simulink model "AutonomousCleaningSystem"  (R2022b)
settings: Solver=VariableStepAuto  StartTime=0.0  StopTime=10.0  RelTol=1e-3
undefined symbols (not defined in the file): Camera_data, Lidar
settings Model: Creator=carol  LastModifiedBy=carol
settings OptimizationCC: ReuseModelBlockBuffer=on

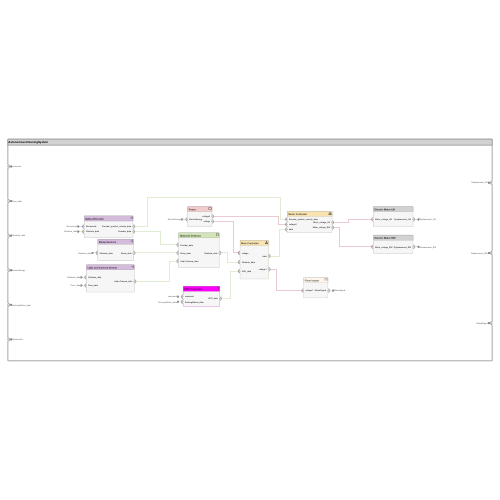
[thumbnail: Simulink's stored preview of the top-level diagram]
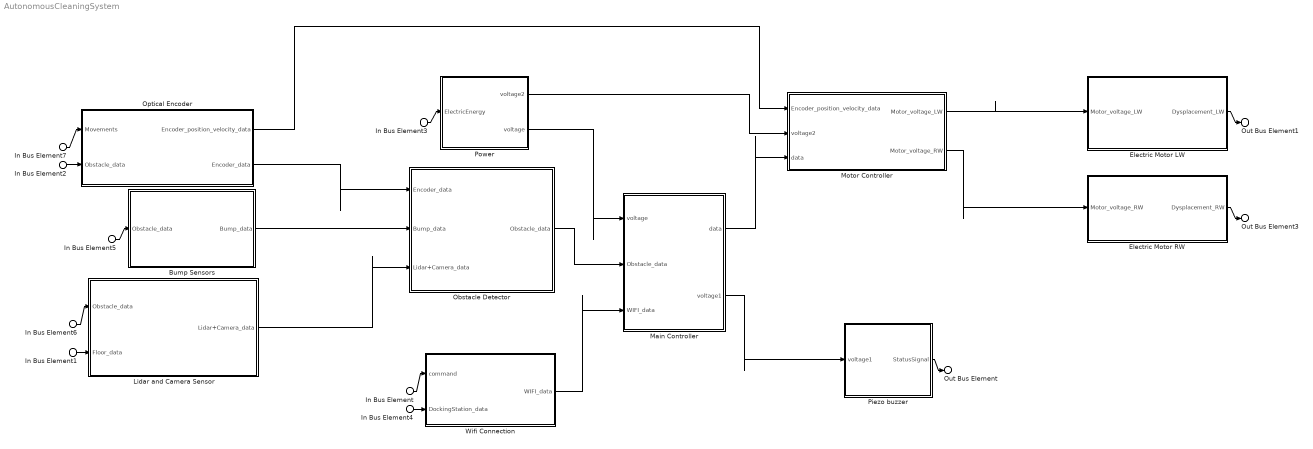
== system AutonomousCleaningSystem ==
  In Bus Element : Inport  PortName=command
  In Bus Element1 : Inport  Port=2  PortName=Floor_data
  In Bus Element2 : Inport  Port=3  PortName=Obstacle_data
  In Bus Element5 : Inport  Port=3  PortName=Obstacle_data
  In Bus Element6 : Inport  Port=3  PortName=Obstacle_data
  In Bus Element3 : Inport  Port=4  PortName=ElectricEnergy
  In Bus Element4 : Inport  Port=5  PortName=DockingStation_data
  In Bus Element7 : Inport  Port=6  PortName=Movements
  Bump Sensors : Subsystem
      settings: PortSchema="{\"entries\":[{\"content\":{\"headerSize\":26,\"margin\":15,\"minimumSpacing\":25,\"sides\":[{\"content\":{\"connectorIds\":[\"In1\"]},\"type\":\"ConnectorPlacement.EquallySpacedRectSide\",\"uuid\":\"6ae6270c-bff4-4a0d-8fba-8fdec87b0a05\"},{\"content\":{\"connectorIds\":[\"Out1\"],\"side\":\"RIGHT\"},\"type\":\"ConnectorPlacement.EquallySpacedRectSide\",\"uuid\":\"f3a0045b-bb3b-40f9-afd5-e1537ff3eeca\"},{\"content\":{\"side\":\"TOP\"},\"type\":\"ConnectorPlacement.EquallySpacedRectSide\",\"uuid\":\"e89a58f2-90b0-468c-bb6a-95617af68e24\"}]},\"type\":\"ConnectorPlacement.EquallySpacedConnector\",\"uuid\":\"066eb43c-7b96-4660-9f29-628dd77a5b3b\"}],\"packageUris\":[\"http://schema.mathworks.com/mf0/Connector/R2020b\"],\"version\":\"1.0\"}"
  Electric Motor LW : Subsystem
      settings: PortSchema="{\"entries\":[{\"content\":{\"headerSize\":26,\"margin\":15,\"minimumSpacing\":25,\"sides\":[{\"content\":{\"connectorIds\":[\"In1\"]},\"type\":\"ConnectorPlacement.EquallySpacedRectSide\",\"uuid\":\"6ae6270c-bff4-4a0d-8fba-8fdec87b0a05\"},{\"content\":{\"connectorIds\":[\"Out1\"],\"side\":\"RIGHT\"},\"type\":\"ConnectorPlacement.EquallySpacedRectSide\",\"uuid\":\"f3a0045b-bb3b-40f9-afd5-e1537ff3eeca\"},{\"content\":{\"side\":\"TOP\"},\"type\":\"ConnectorPlacement.EquallySpacedRectSide\",\"uuid\":\"e89a58f2-90b0-468c-bb6a-95617af68e24\"}]},\"type\":\"ConnectorPlacement.EquallySpacedConnector\",\"uuid\":\"066eb43c-7b96-4660-9f29-628dd77a5b3b\"}],\"packageUris\":[\"http://schema.mathworks.com/mf0/Connector/R2020b\"],\"version\":\"1.0\"}"
  Electric Motor RW : Subsystem
      settings: PortSchema="{\"entries\":[{\"content\":{\"headerSize\":26,\"margin\":15,\"minimumSpacing\":25,\"sides\":[{\"content\":{\"connectorIds\":[\"In1\"]},\"type\":\"ConnectorPlacement.EquallySpacedRectSide\",\"uuid\":\"6ae6270c-bff4-4a0d-8fba-8fdec87b0a05\"},{\"content\":{\"connectorIds\":[\"Out1\"],\"side\":\"RIGHT\"},\"type\":\"ConnectorPlacement.EquallySpacedRectSide\",\"uuid\":\"f3a0045b-bb3b-40f9-afd5-e1537ff3eeca\"},{\"content\":{\"side\":\"TOP\"},\"type\":\"ConnectorPlacement.EquallySpacedRectSide\",\"uuid\":\"e89a58f2-90b0-468c-bb6a-95617af68e24\"}]},\"type\":\"ConnectorPlacement.EquallySpacedConnector\",\"uuid\":\"066eb43c-7b96-4660-9f29-628dd77a5b3b\"}],\"packageUris\":[\"http://schema.mathworks.com/mf0/Connector/R2020b\"],\"version\":\"1.0\"}"
  Lidar and Camera Sensor : Subsystem
      settings: PortSchema="{\"entries\":[{\"content\":{\"headerSize\":26,\"margin\":15,\"minimumSpacing\":25,\"sides\":[{\"content\":{\"connectorIds\":[\"In1\",\"In2\"]},\"type\":\"ConnectorPlacement.EquallySpacedRectSide\",\"uuid\":\"6ae6270c-bff4-4a0d-8fba-8fdec87b0a05\"},{\"content\":{\"connectorIds\":[\"Out1\"],\"side\":\"RIGHT\"},\"type\":\"ConnectorPlacement.EquallySpacedRectSide\",\"uuid\":\"f3a0045b-bb3b-40f9-afd5-e1537ff3eeca\"},{\"content\":{\"side\":\"TOP\"},\"type\":\"ConnectorPlacement.EquallySpacedRectSide\",\"uuid\":\"e89a58f2-90b0-468c-bb6a-95617af68e24\"}]},\"type\":\"ConnectorPlacement.EquallySpacedConnector\",\"uuid\":\"066eb43c-7b96-4660-9f29-628dd77a5b3b\"}],\"packageUris\":[\"http://schema.mathworks.com/mf0/Connector/R2020b\"],\"version\":\"1.0\"}"
  Main Controller : Subsystem
      settings: PortSchema="{\"entries\":[{\"content\":{\"headerSize\":26,\"margin\":15,\"minimumSpacing\":25,\"sides\":[{\"content\":{\"connectorIds\":[\"In1\",\"In2\",\"In3\"]},\"type\":\"ConnectorPlacement.EquallySpacedRectSide\",\"uuid\":\"6ae6270c-bff4-4a0d-8fba-8fdec87b0a05\"},{\"content\":{\"connectorIds\":[\"Out1\",\"Out2\"],\"side\":\"RIGHT\"},\"type\":\"ConnectorPlacement.EquallySpacedRectSide\",\"uuid\":\"f3a0045b-bb3b-40f9-afd5-e1537ff3eeca\"},{\"content\":{\"side\":\"TOP\"},\"type\":\"ConnectorPlacement.EquallySpacedRectSide\",\"uuid\":\"e89a58f2-90b0-468c-bb6a-95617af68e24\"}]},\"type\":\"ConnectorPlacement.EquallySpacedConnector\",\"uuid\":\"066eb43c-7b96-4660-9f29-628dd77a5b3b\"}],\"packageUris\":[\"http://schema.mathworks.com/mf0/Connector/R2020b\"],\"version\":\"1.0\"}"
  Motor Controller : Subsystem
      settings: PortSchema="{\"entries\":[{\"content\":{\"headerSize\":26,\"margin\":15,\"minimumSpacing\":25,\"sides\":[{\"content\":{\"connectorIds\":[\"In1\",\"In2\",\"In3\"]},\"type\":\"ConnectorPlacement.EquallySpacedRectSide\",\"uuid\":\"6ae6270c-bff4-4a0d-8fba-8fdec87b0a05\"},{\"content\":{\"connectorIds\":[\"Out1\",\"Out2\"],\"side\":\"RIGHT\"},\"type\":\"ConnectorPlacement.EquallySpacedRectSide\",\"uuid\":\"f3a0045b-bb3b-40f9-afd5-e1537ff3eeca\"},{\"content\":{\"side\":\"TOP\"},\"type\":\"ConnectorPlacement.EquallySpacedRectSide\",\"uuid\":\"e89a58f2-90b0-468c-bb6a-95617af68e24\"}]},\"type\":\"ConnectorPlacement.EquallySpacedConnector\",\"uuid\":\"066eb43c-7b96-4660-9f29-628dd77a5b3b\"}],\"packageUris\":[\"http://schema.mathworks.com/mf0/Connector/R2020b\"],\"version\":\"1.0\"}"
  Obstacle Detector : Subsystem
      settings: PortSchema="{\"entries\":[{\"content\":{\"headerSize\":26,\"margin\":15,\"minimumSpacing\":25,\"sides\":[{\"content\":{\"connectorIds\":[\"In1\",\"In2\",\"In3\"]},\"type\":\"ConnectorPlacement.EquallySpacedRectSide\",\"uuid\":\"6ae6270c-bff4-4a0d-8fba-8fdec87b0a05\"},{\"content\":{\"connectorIds\":[\"Out1\"],\"side\":\"RIGHT\"},\"type\":\"ConnectorPlacement.EquallySpacedRectSide\",\"uuid\":\"f3a0045b-bb3b-40f9-afd5-e1537ff3eeca\"},{\"content\":{\"side\":\"TOP\"},\"type\":\"ConnectorPlacement.EquallySpacedRectSide\",\"uuid\":\"e89a58f2-90b0-468c-bb6a-95617af68e24\"}]},\"type\":\"ConnectorPlacement.EquallySpacedConnector\",\"uuid\":\"066eb43c-7b96-4660-9f29-628dd77a5b3b\"}],\"packageUris\":[\"http://schema.mathworks.com/mf0/Connector/R2020b\"],\"version\":\"1.0\"}"
  Optical Encoder : Subsystem
      settings: PortSchema="{\"entries\":[{\"content\":{\"headerSize\":26,\"margin\":15,\"minimumSpacing\":25,\"sides\":[{\"content\":{\"connectorIds\":[\"In1\",\"In2\"]},\"type\":\"ConnectorPlacement.EquallySpacedRectSide\",\"uuid\":\"6ae6270c-bff4-4a0d-8fba-8fdec87b0a05\"},{\"content\":{\"connectorIds\":[\"Out1\",\"Out2\"],\"side\":\"RIGHT\"},\"type\":\"ConnectorPlacement.EquallySpacedRectSide\",\"uuid\":\"f3a0045b-bb3b-40f9-afd5-e1537ff3eeca\"},{\"content\":{\"side\":\"TOP\"},\"type\":\"ConnectorPlacement.EquallySpacedRectSide\",\"uuid\":\"e89a58f2-90b0-468c-bb6a-95617af68e24\"}]},\"type\":\"ConnectorPlacement.EquallySpacedConnector\",\"uuid\":\"066eb43c-7b96-4660-9f29-628dd77a5b3b\"}],\"packageUris\":[\"http://schema.mathworks.com/mf0/Connector/R2020b\"],\"version\":\"1.0\"}"
  Piezo buzzer : Subsystem
      settings: PortSchema="{\"entries\":[{\"content\":{\"headerSize\":26,\"margin\":15,\"minimumSpacing\":25,\"sides\":[{\"content\":{\"connectorIds\":[\"In1\"]},\"type\":\"ConnectorPlacement.EquallySpacedRectSide\",\"uuid\":\"6ae6270c-bff4-4a0d-8fba-8fdec87b0a05\"},{\"content\":{\"connectorIds\":[\"Out1\"],\"side\":\"RIGHT\"},\"type\":\"ConnectorPlacement.EquallySpacedRectSide\",\"uuid\":\"f3a0045b-bb3b-40f9-afd5-e1537ff3eeca\"},{\"content\":{\"side\":\"TOP\"},\"type\":\"ConnectorPlacement.EquallySpacedRectSide\",\"uuid\":\"e89a58f2-90b0-468c-bb6a-95617af68e24\"}]},\"type\":\"ConnectorPlacement.EquallySpacedConnector\",\"uuid\":\"066eb43c-7b96-4660-9f29-628dd77a5b3b\"}],\"packageUris\":[\"http://schema.mathworks.com/mf0/Connector/R2020b\"],\"version\":\"1.0\"}"
  Power : Subsystem
      settings: PortSchema="{\"entries\":[{\"content\":{\"headerSize\":26,\"margin\":15,\"minimumSpacing\":25,\"sides\":[{\"content\":{\"connectorIds\":[\"In1\"]},\"type\":\"ConnectorPlacement.EquallySpacedRectSide\",\"uuid\":\"6ae6270c-bff4-4a0d-8fba-8fdec87b0a05\"},{\"content\":{\"connectorIds\":[\"Out2\",\"Out1\"],\"side\":\"RIGHT\"},\"type\":\"ConnectorPlacement.EquallySpacedRectSide\",\"uuid\":\"f3a0045b-bb3b-40f9-afd5-e1537ff3eeca\"},{\"content\":{\"side\":\"TOP\"},\"type\":\"ConnectorPlacement.EquallySpacedRectSide\",\"uuid\":\"e89a58f2-90b0-468c-bb6a-95617af68e24\"}]},\"type\":\"ConnectorPlacement.EquallySpacedConnector\",\"uuid\":\"066eb43c-7b96-4660-9f29-628dd77a5b3b\"}],\"packageUris\":[\"http://schema.mathworks.com/mf0/Connector/R2020b\"],\"version\":\"1.0\"}"
  Wifi Connection : Subsystem
      settings: PortSchema="{\"entries\":[{\"content\":{\"headerSize\":26,\"margin\":15,\"minimumSpacing\":25,\"sides\":[{\"content\":{\"connectorIds\":[\"In2\",\"In1\"]},\"type\":\"ConnectorPlacement.EquallySpacedRectSide\",\"uuid\":\"6ae6270c-bff4-4a0d-8fba-8fdec87b0a05\"},{\"content\":{\"connectorIds\":[\"Out1\"],\"side\":\"RIGHT\"},\"type\":\"ConnectorPlacement.EquallySpacedRectSide\",\"uuid\":\"f3a0045b-bb3b-40f9-afd5-e1537ff3eeca\"},{\"content\":{\"side\":\"TOP\"},\"type\":\"ConnectorPlacement.EquallySpacedRectSide\",\"uuid\":\"e89a58f2-90b0-468c-bb6a-95617af68e24\"}]},\"type\":\"ConnectorPlacement.EquallySpacedConnector\",\"uuid\":\"066eb43c-7b96-4660-9f29-628dd77a5b3b\"}],\"packageUris\":[\"http://schema.mathworks.com/mf0/Connector/R2020b\"],\"version\":\"1.0\"}"
  Out Bus Element1 : Outport  PortName=Displacement_LW
  Out Bus Element3 : Outport  Port=2  PortName=Displacement_RW
  Out Bus Element : Outport  Port=3  PortName=StatusSignal
  wires:
  In Bus Element4/1 -> Wifi Connection/1(DockingStation_data)
  Obstacle Detector/1(Obstacle_data) -> Main Controller/2(Obstacle_data)
  Electric Motor LW/1(Dysplacement_LW) -> Out Bus Element1/1
  Piezo buzzer/1(StatusSignal) -> Out Bus Element/1
  In Bus Element1/1 -> Lidar and Camera Sensor/2(Floor_data)
  Electric Motor RW/1(Dysplacement_RW) -> Out Bus Element3/1
  Wifi Connection/1(WIFI_data) -> Main Controller/3(WIFI_data)
  In Bus Element7/1 -> Optical Encoder/1(Movements)
  Motor Controller/2(Motor_voltage_RW) -> Electric Motor RW/1(Motor_voltage_RW)
  In Bus Element/1 -> Wifi Connection/2(command)
  Power/1(voltage) -> Main Controller/1(voltage)
  In Bus Element3/1 -> Power/1(ElectricEnergy)
  In Bus Element2/1 -> Optical Encoder/2(Obstacle_data)
  Optical Encoder/2(Encoder_data) -> Obstacle Detector/1(Encoder_data)
  Main Controller/2(voltage1) -> Piezo buzzer/1(voltage1)
  Motor Controller/1(Motor_voltage_LW) -> Electric Motor LW/1(Motor_voltage_LW)
  In Bus Element6/1 -> Lidar and Camera Sensor/1(Obstacle_data)
  In Bus Element5/1 -> Bump Sensors/1(Obstacle_data)
  Main Controller/1(data) -> Motor Controller/3(data)
  Optical Encoder/1(Encoder_position_velocity_data) -> Motor Controller/1(Encoder_position_velocity_data)
  Bump Sensors/1(Bump_data) -> Obstacle Detector/2(Bump_data)
  Lidar and Camera Sensor/1(Lidar+Camera_data) -> Obstacle Detector/3(Lidar+Camera_data)
  Power/2(voltage2) -> Motor Controller/2(voltage2)

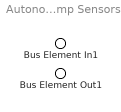
== system AutonomousCleaningSystem/Bump Sensors ==
  Bus Element In1 : Inport  PortName=Obstacle_data
  Bus Element Out1 : Outport  PortName=Bump_data

== system AutonomousCleaningSystem/Electric Motor LW ==
  Bus Element In1 : Inport  PortName=Motor_voltage_LW
  Bus Element Out1 : Outport  PortName=Dysplacement_LW

== system AutonomousCleaningSystem/Electric Motor RW ==
  Bus Element In1 : Inport  PortName=Motor_voltage_RW
  Bus Element Out1 : Outport  PortName=Dysplacement_RW

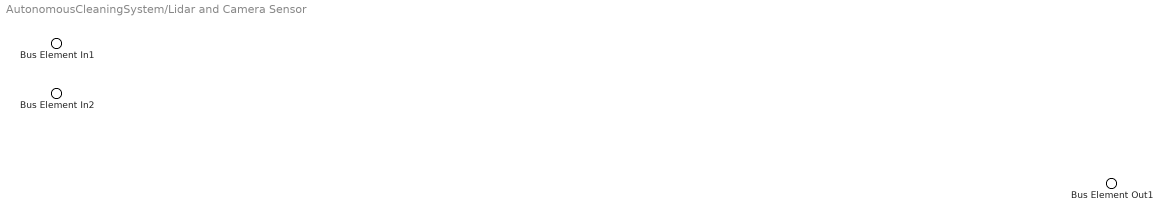
== system AutonomousCleaningSystem/Lidar and Camera Sensor ==
  Bus Element In1 : Inport  PortName=Obstacle_data
  Bus Element In2 : Inport  Port=2  PortName=Floor_data
  Bus Element Out1 : Outport  PortName=Lidar+Camera_data

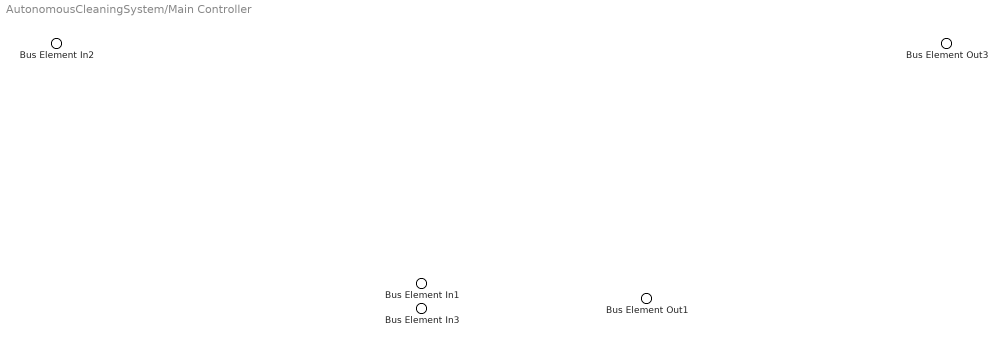
== system AutonomousCleaningSystem/Main Controller ==
  Bus Element In2 : Inport  PortName=voltage
  Bus Element In1 : Inport  Port=2  PortName=Obstacle_data
  Bus Element In3 : Inport  Port=3  PortName=WIFI_data
  Bus Element Out1 : Outport  PortName=data
  Bus Element Out3 : Outport  Port=2  PortName=voltage1

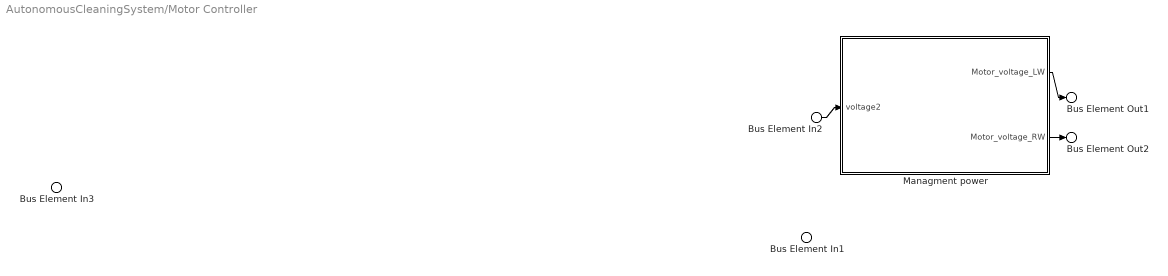
== system AutonomousCleaningSystem/Motor Controller ==
  Bus Element In3 : Inport  PortName=Encoder_position_velocity_data
  Bus Element In2 : Inport  Port=2  PortName=voltage2
  Bus Element In1 : Inport  Port=3  PortName=data
  Managment power : Subsystem
      settings: PortSchema="{\"entries\":[{\"content\":{\"headerSize\":26,\"margin\":15,\"minimumSpacing\":25,\"sides\":[{\"content\":{\"connectorIds\":[\"In1\"]},\"type\":\"ConnectorPlacement.EquallySpacedRectSide\",\"uuid\":\"8bc022de-dffb-4362-a5f8-17ef95234df5\"},{\"content\":{\"connectorIds\":[\"Out1\",\"Out2\"],\"side\":\"RIGHT\"},\"type\":\"ConnectorPlacement.EquallySpacedRectSide\",\"uuid\":\"7821fee0-4f8e-4fbb-ae89-26aabe366038\"},{\"content\":{\"side\":\"TOP\"},\"type\":\"ConnectorPlacement.EquallySpacedRectSide\",\"uuid\":\"eaa51f63-b7e5-4e12-92d3-5116fe88bdcc\"}]},\"type\":\"ConnectorPlacement.EquallySpacedConnector\",\"uuid\":\"a20c8fba-198d-4ab4-9322-4dfa42a9e59c\"}],\"packageUris\":[\"http://schema.mathworks.com/mf0/Connector/R2020b\"],\"version\":\"1.0\"}"
  Bus Element Out1 : Outport  PortName=Motor_voltage_LW
  Bus Element Out2 : Outport  Port=2  PortName=Motor_voltage_RW
  wires:
  Bus Element In2/1 -> Managment power/1(voltage2)
  Managment power/1(Motor_voltage_LW) -> Bus Element Out1/1
  Managment power/2(Motor_voltage_RW) -> Bus Element Out2/1

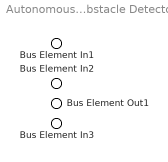
== system AutonomousCleaningSystem/Obstacle Detector ==
  Bus Element In1 : Inport  PortName=Encoder_data
  Bus Element In2 : Inport  Port=2  PortName=Bump_data
  Bus Element In3 : Inport  Port=3  PortName=Lidar+Camera_data
  Bus Element Out1 : Outport  PortName=Obstacle_data

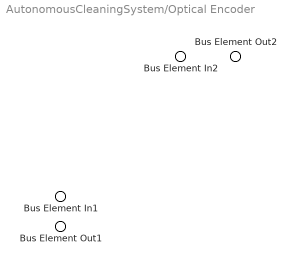
== system AutonomousCleaningSystem/Optical Encoder ==
  Bus Element In2 : Inport  PortName=Movements
  Bus Element In1 : Inport  Port=2  PortName=Obstacle_data
  Bus Element Out2 : Outport  PortName=Encoder_position_velocity_data
  Bus Element Out1 : Outport  Port=2  PortName=Encoder_data

== system AutonomousCleaningSystem/Piezo buzzer ==
  Bus Element In1 : Inport  PortName=voltage1
  Bus Element Out1 : Outport  PortName=StatusSignal

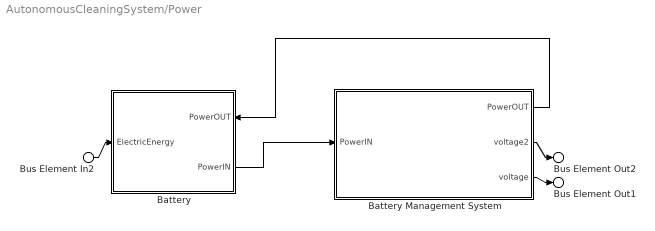
== system AutonomousCleaningSystem/Power ==
  Bus Element In2 : Inport  PortName=ElectricEnergy
  Battery : Subsystem
      settings: PortSchema="{\"entries\":[{\"content\":{\"headerSize\":26,\"margin\":15,\"minimumSpacing\":25,\"sides\":[{\"content\":{\"connectorIds\":[\"In2\"]},\"type\":\"ConnectorPlacement.EquallySpacedRectSide\",\"uuid\":\"8bc022de-dffb-4362-a5f8-17ef95234df5\"},{\"content\":{\"connectorIds\":[\"In1\",\"Out1\"],\"side\":\"RIGHT\"},\"type\":\"ConnectorPlacement.EquallySpacedRectSide\",\"uuid\":\"7821fee0-4f8e-4fbb-ae89-26aabe366038\"},{\"content\":{\"side\":\"TOP\"},\"type\":\"ConnectorPlacement.EquallySpacedRectSide\",\"uuid\":\"eaa51f63-b7e5-4e12-92d3-5116fe88bdcc\"}]},\"type\":\"ConnectorPlacement.EquallySpacedConnector\",\"uuid\":\"a20c8fba-198d-4ab4-9322-4dfa42a9e59c\"}],\"packageUris\":[\"http://schema.mathworks.com/mf0/Connector/R2020b\"],\"version\":\"1.0\"}"
  Battery Management System : Subsystem
      settings: PortSchema="{\"entries\":[{\"content\":{\"headerSize\":26,\"margin\":15,\"minimumSpacing\":25,\"sides\":[{\"content\":{\"connectorIds\":[\"In1\"]},\"type\":\"ConnectorPlacement.EquallySpacedRectSide\",\"uuid\":\"8bc022de-dffb-4362-a5f8-17ef95234df5\"},{\"content\":{\"connectorIds\":[\"Out1\",\"Out2\",\"Out3\"],\"side\":\"RIGHT\"},\"type\":\"ConnectorPlacement.EquallySpacedRectSide\",\"uuid\":\"7821fee0-4f8e-4fbb-ae89-26aabe366038\"},{\"content\":{\"side\":\"TOP\"},\"type\":\"ConnectorPlacement.EquallySpacedRectSide\",\"uuid\":\"eaa51f63-b7e5-4e12-92d3-5116fe88bdcc\"}]},\"type\":\"ConnectorPlacement.EquallySpacedConnector\",\"uuid\":\"a20c8fba-198d-4ab4-9322-4dfa42a9e59c\"}],\"packageUris\":[\"http://schema.mathworks.com/mf0/Connector/R2020b\"],\"version\":\"1.0\"}"
  Bus Element Out1 : Outport  PortName=voltage
  Bus Element Out2 : Outport  Port=2  PortName=voltage2
  wires:
  Battery/1(PowerIN) -> Battery Management System/1(PowerIN)
  Bus Element In2/1 -> Battery/2(ElectricEnergy)
  Battery Management System/1(PowerOUT) -> Battery/1(PowerOUT)
  Battery Management System/2(voltage2) -> Bus Element Out2/1
  Battery Management System/3(voltage) -> Bus Element Out1/1

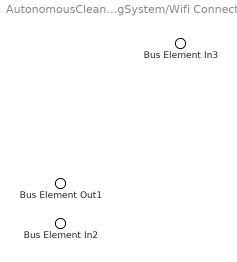
== system AutonomousCleaningSystem/Wifi Connection ==
  Bus Element In3 : Inport  PortName=DockingStation_data
  Bus Element In2 : Inport  Port=2  PortName=command
  Bus Element Out1 : Outport  PortName=WIFI_data

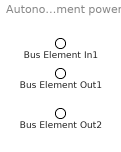
== system AutonomousCleaningSystem/Motor Controller/Managment power ==
  Bus Element In1 : Inport  PortName=voltage2
  Bus Element Out1 : Outport  PortName=Motor_voltage_LW
  Bus Element Out2 : Outport  Port=2  PortName=Motor_voltage_RW

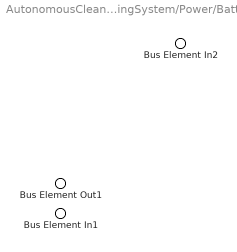
== system AutonomousCleaningSystem/Power/Battery ==
  Bus Element In2 : Inport  PortName=PowerOUT
  Bus Element In1 : Inport  Port=2  PortName=ElectricEnergy
  Bus Element Out1 : Outport  PortName=PowerIN

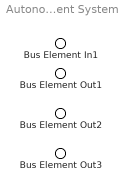
== system AutonomousCleaningSystem/Power/Battery Management System ==
  Bus Element In1 : Inport  PortName=PowerIN
  Bus Element Out1 : Outport  PortName=PowerOUT
  Bus Element Out2 : Outport  Port=2  PortName=voltage2
  Bus Element Out3 : Outport  Port=3  PortName=voltage
